simulink model "Half_car_roll"  (R2024b)
settings: Solver=VariableStepAuto  StartTime=0.0  StopTime=10.0  RelTol=1e-3
undefined symbols (not defined in the file): Af, Cf_sprung, Cl, Kf_sprung, Kf_unsprung, M_sprung, Mf_unsprung, Mr_unsprung, rho, tw_front
settings Model: Creator=kanishka  LastModifiedBy=kanishka

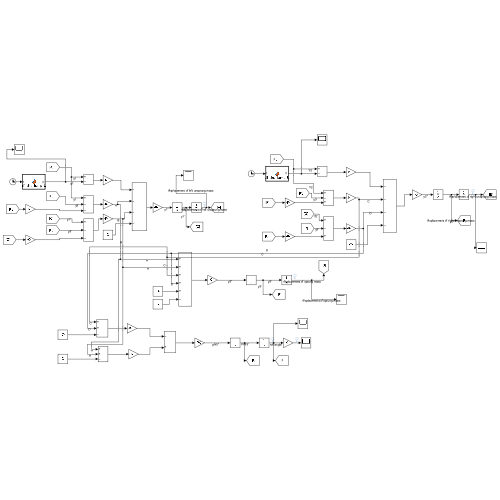
[thumbnail: Simulink's stored preview of the top-level diagram]
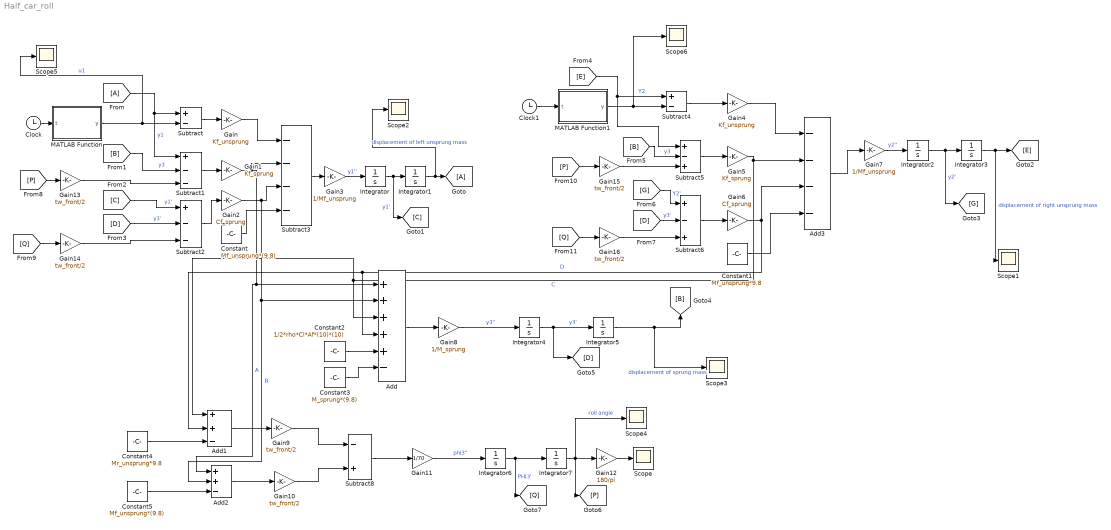
== system Half_car_roll ==
  Add : Sum  Inputs=+++++-
  Add1 : Sum  Inputs=++-
  Add2 : Sum  Inputs=++-
  Add3 : Sum  Inputs=----
  Clock : Clock
  Clock1 : Clock
  Constant : Constant  Value=Mf_unsprung*(9.8)
  Constant1 : Constant  Value=Mf_unsprung*9.8
  Constant2 : Constant  Value=1/2*rho*Cl*Af*(10)*(10)
  Constant3 : Constant  Value=M_sprung*(9.8)
  Constant4 : Constant  Value=Mr_unsprung*9.8
  Constant5 : Constant  Value=Mf_unsprung*(9.8)
  From : From
  Gain : Gain  Gain=Kf_unsprung
  Gain1 : Gain  Gain=Kf_sprung
  Gain{9..10,13..16} (6 alike) : Gain  Gain=tw_front/2
  Gain11 : Gain  Gain=1/70
  Gain12 : Gain  Gain=180/pi
  Gain2 : Gain  Gain=Cf_sprung
  Gain3 : Gain  Gain=1/Mf_unsprung
  Gain4 : Gain  Gain=Kf_unsprung
  Gain5 : Gain  Gain=Kf_sprung
  Gain6 : Gain  Gain=Cf_sprung
  Gain7 : Gain  Gain=1/Mf_unsprung
  Gain8 : Gain  Gain=1/M_sprung
  Goto : Goto
  Integrator{,1..7} (8 alike) : Integrator
  MATLAB Function : MATLAB Function  TreatAsAtomicUnit=on
  MATLAB Function1 : MATLAB Function  TreatAsAtomicUnit=on
  Scope{,1..6} (7 alike) : Scope
  Subtract : Sum  Inputs=+-
  Subtract1 : Sum  Inputs=+--
  Subtract2 : Sum  Inputs=+--
  Subtract3 : Sum  Inputs=----
  Subtract4 : Sum  Inputs=+-
  Subtract5 : Sum  Inputs=+-+
  Subtract6 : Sum  Inputs=+-+
  Subtract8 : Sum  Inputs=-+
  wires:
  Gain/1 -> Subtract3/1
  Constant/1 -> Subtract3/4
  Integrator6/1 -> [Q], Integrator7/1  "PHI3'"
  [D] -> Subtract6/2  "y3'"
  Subtract5/1 -> Gain5/1
  Constant2/1 -> Add/5
  Subtract8/1 -> Gain11/1
  Subtract2/1 -> Gain2/1
  Gain9/1 -> Subtract8/1
  Gain8/1 -> Integrator4/1  "y3''"
  Subtract6/1 -> Gain6/1
  Constant3/1 -> Add/6
  Gain13/1 -> Subtract1/3
  [B] -> Subtract1/2  "y3"
  Integrator1/1 -> Scope2/1, Goto/1  "displacement of left unsprung mass"
  Gain10/1 -> Subtract8/2
  [C] -> Subtract2/1  "y1'"
  MATLAB Function1/1(y) -> Scope6/1, Subtract4/2
  Gain11/1 -> Integrator6/1  "phi3''"
  Add2/1 -> Gain10/1
  Gain14/1 -> Subtract2/3
  Integrator4/1 -> [D], Integrator5/1  "y3'"
  [Q] -> Gain14/1
  Gain1/1 -> Subtract3/2, Add2/1, Add/1  "A"
  Gain4/1 -> Add3/1
  Add/1 -> Gain8/1
  Integrator7/1 -> Scope4/1, [P], Gain12/1  "roll angle"
  Clock/1 -> MATLAB Function/1(t)
  Gain3/1 -> Integrator/1  "y1''"
  [Q] -> Gain16/1
  Subtract1/1 -> Gain1/1
  Gain2/1 -> Subtract3/3, Add/2, Add2/2  "B"
  Gain7/1 -> Integrator2/1  "y2''"
  Constant1/1 -> Add3/4
  From/1 -> Subtract1/1, Subtract/1  "y1"
  Gain16/1 -> Subtract6/3
  Add1/1 -> Gain9/1
  [D] -> Subtract2/2  "y3'"
  Integrator5/1 -> Scope3/1, [B]  "displacement of sprung mass"
  Subtract4/1 -> Gain4/1
  MATLAB Function/1(y) -> Scope5/1, Subtract/2  "u1"
  [B] -> Subtract5/2  "y3"
  Subtract3/1 -> Gain3/1
  Constant5/1 -> Add2/3
  Gain5/1 -> Add3/2, Add1/1, Add/3  "C"
  [P] -> Gain15/1
  Clock1/1 -> MATLAB Function1/1(t)
  Gain12/1 -> Scope/1
  Gain6/1 -> Add3/3, Add1/2, Add/4  "D"
  [G] -> Subtract6/1  "Y2'"
  [E] -> Subtract4/1, Subtract5/1  "Y2"
  Constant4/1 -> Add1/3
  Integrator3/1 -> [E], Scope1/1  "displacement of right unsprung mass"
  Integrator/1 -> [C], Integrator1/1  "y1'"
  Add3/1 -> Gain7/1
  [P] -> Gain13/1
  Subtract/1 -> Gain/1
  Integrator2/1 -> Integrator3/1, [G]  "y2'"
  Gain15/1 -> Subtract5/3

== matlab function Half_car_roll/MATLAB Function ==
  data: t input; y output
function y = half_sine_bump_U1(t)

amplitude = 0.05;     
wavelength = 0.6;      
v = 10;                


x = v * t;

% Generate half sine wave profile for 0 <= x <= 0.3
if x >= 0 && x <= wavelength/2
    y = amplitude * sin((2*pi * x) / wavelength);
else
    y = 0;
end
end

== matlab function Half_car_roll/MATLAB Function1 ==
  data: t input; y output
function y = half_sine_bump_U2(t)
amplitude = 0.05;     
wavelength = 0.6;      
v = 10;                
L = 1.53;             
delay = L / v;


x = v * (t - delay);


if x >= 0 && x <= wavelength/2
    y = amplitude * sin((2*pi * x) / wavelength);
else
    y = 0;
end
end
